simulink model "AsyncOnlinePlanning"  (R2025a)
settings: Solver=FixedStepAuto  StartTime=0.0  StopTime=inf  FixedStep=0.01  RelTol=1e-3  EnableMultiTasking=on
undefined symbols (not defined in the file): enable, finalPose, initialStateAndInput, originLLA, reset, samplingBoxCenterPose, samplingBoxDimension, sequentialPlanner, timestamp, verticesStaticObstacles
libraries: MPSV x4, simulink x2
settings Model: Creator=damerius  LastModifiedBy=damerius
settings SolverCC: ConcurrentTasks=on  AlgebraicLoopSolver=TrustRegion  PositivePriorityOrder=on
settings DataIOCC: SaveOutput=off  SignalLogging=off  DSMLogging=off  SaveTime=off  ReturnWorkspaceOutputs=off
settings OptimizationCC: DefaultParameterBehavior=Inlined  ReuseModelBlockBuffer=off  ZeroExternalMemoryAtStartup=off  ZeroInternalMemoryAtStartup=off  SimCompilerOptimization=on
settings DebuggingCC: UnconnectedInputMsg=warning  UnconnectedOutputMsg=warning  UnconnectedLineMsg=warning
settings HardwareCC: ProdBitPerLong=64.0  ProdHWDeviceType=Intel->x86-64 (Linux 64)
settings ModelReferenceCC: EnableRefExpFcnMdlSchedulingChecks=on
settings SFSimCC: SimParseCustomCode=off  SimGenImportedTypeDefs=on  SimTargetLang=C++  SimDLTargetLibrary=mkl-dnn
settings RTWCC: GenCodeOnly=on  PackageGeneratedCodeAndArtifacts=on  PackageName=PackNGo  RTWVerbose=off  BuildConfiguration=Faster Runs  TargetLang=C++  GPUComputeCapability=3.5  DLArmComputeVersion=19.05
settings CodeAppCC: ForceParamTrailComments=on  MaxIdLength=95.0  MATLABSourceComments=on  UseSimReservedNames=on
settings GRTTargetCC: TargetLangStandard=C++11 (ISO)  GenerateFullHeader=off  MatFileLogging=off  CodeInterfacePackaging=C++ class  SubcomponentCodeInterfacePackaging=C++ class

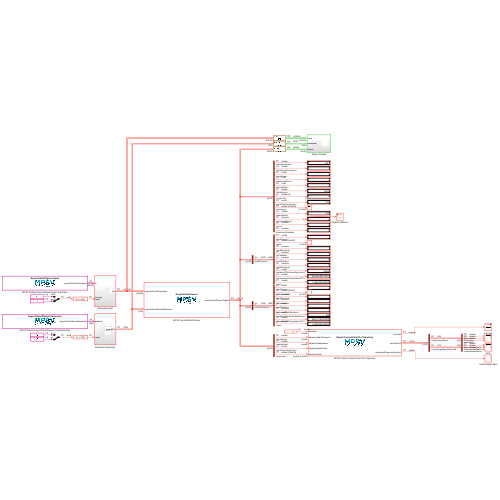
[thumbnail: Simulink's stored preview of the top-level diagram]
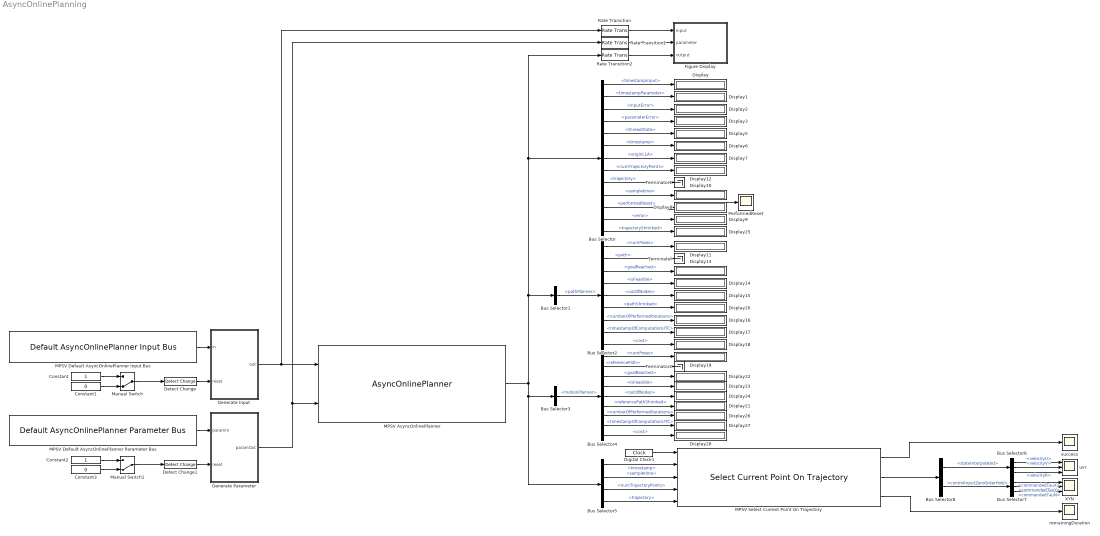
== system AsyncOnlinePlanning ==
  Bus Selector : BusSelector  OutputSignals=timestampInput,timestampParameter,inputError,parameterError,threadState,timestamp,originLLA,numTrajectoryPoints,trajectory,sampletime,performedReset,error,trajectoryShrinked
  Bus Selector1 : BusSelector  OutputSignals=pathPlanner
  Bus Selector2 : BusSelector  OutputSignals=numPoses,path,goalReached,isFeasible,outOfNodes,pathShrinked,numberOfPerformedIterations,timestampOfComputationUTC,cost
  Bus Selector3 : BusSelector  OutputSignals=motionPlanner
  Bus Selector4 : BusSelector  OutputSignals=numPoses,referencePath,goalReached,isFeasible,outOfNodes,referencePathShrinked,numberOfPerformedIterations,timestampOfComputationUTC,cost
  Bus Selector5 : BusSelector  OutputSignals=timestamp,sampletime,numTrajectoryPoints,trajectory
  Bus Selector6 : BusSelector  OutputSignals=velocityU,velocityV,velocityR
  Bus Selector7 : BusSelector  OutputSignals=commandedTauX,commandedTauY,commandedTauN
  Bus Selector8 : BusSelector  OutputSignals=stateInterpolated,controlInputZeroOrderHold
  Constant : Constant  OutDataTypeStr=uint8
  Constant1 : Constant  Value=0  OutDataTypeStr=uint8
  Constant2 : Constant  OutDataTypeStr=uint8
  Constant3 : Constant  Value=0  OutDataTypeStr=uint8
  Detect Change : simulink/Logic and Bit Operations/Detect Change  vinit=0  OutDataTypeStr=boolean
  Detect Change1 : simulink/Logic and Bit Operations/Detect Change  vinit=0  OutDataTypeStr=boolean
  Digital Clock1 : DigitalClock  SampleTime=0.01
  Display{,1..3,5..28} (28 alike) : Display
  Figure Display : Subsystem
  Generate Input : Subsystem
  Generate Parameter : Subsystem
  MPSV AsyncOnlinePlanner : MPSV/AsyncOnlinePlanner  pathMaxNumNodes=250  pathMaxNumSamples=1000000  motionMaxNumNodes=250  motionMaxNumSamples=1000000  threadPriority=20  cpuCoreIDs=[]  ompNumThreads=-1  ompDynamic=-1
      settings: SourceProductName=MPSV - Motion Planner for Surface Vehicles
  MPSV Default AsyncOnlinePlanner Input Bus : MPSV/Default AsyncOnlinePlanner Input Bus
      settings: SourceProductName=MPSV - Motion Planner for Surface Vehicles
  MPSV Default AsyncOnlinePlanner Parameter Bus : MPSV/Default AsyncOnlinePlanner Parameter Bus
      settings: SourceProductName=MPSV - Motion Planner for Surface Vehicles
  MPSV Select Current Point On Trajectory : MPSV/Select Current Point On Trajectory
      settings: SourceProductName=MPSV - Motion Planner for Surface Vehicles
  Manual Switch : ManualSwitch  CurrentSetting=0
  Manual Switch1 : ManualSwitch  CurrentSetting=0
  PerformedReset : Scope
      settings: ActiveDisplayYMinimum=-0.125  ActiveDisplayYMaximum=1.125
  Rate Transition : RateTransition  Deterministic=off  OutPortSampleTime=1
  Rate Transition1 : RateTransition  Deterministic=off  OutPortSampleTime=1
  Rate Transition2 : RateTransition  Deterministic=off  OutPortSampleTime=1
  Terminator : Terminator
  Terminator1 : Terminator
  Terminator2 : Terminator
  XYN : Scope  NumInputPorts=3
      settings: ActiveDisplayYMinimum=-501.70849  ActiveDisplayYMaximum=735.84406
  remainingDuration : Scope
      settings: ActiveDisplayYMinimum=-2.9925  ActiveDisplayYMaximum=26.9325
  success : Scope
      settings: ActiveDisplayYMinimum=-0.125  ActiveDisplayYMaximum=1.125
  uvr : Scope  NumInputPorts=3
      settings: ActiveDisplayYMinimum=-0.33623  ActiveDisplayYMaximum=0.74355  DataLoggingVariableName=ScopeData2
  wires:
  MPSV Default AsyncOnlinePlanner Parameter Bus/1 -> Generate Parameter/1(paramIn)
  MPSV Default AsyncOnlinePlanner Input Bus/1 -> Generate Input/1(in)
  MPSV AsyncOnlinePlanner/1 -> Bus Selector5/1, Bus Selector3/1, Rate Transition2/1, Bus Selector/1, Bus Selector1/1
  Bus Selector/1 -> Display/1  "<timestampInput>"
  Bus Selector/2 -> Display1/1  "<timestampParameter>"
  Bus Selector/6 -> Display6/1  "<timestamp>"
  Bus Selector/7 -> Display7/1  "<originLLA>"
  Bus Selector/5 -> Display5/1  "<threadState>"
  Bus Selector/12 -> Display9/1  "<error>"
  Bus Selector/11 -> PerformedReset/1, Display8/1  "<performedReset>"
  Generate Parameter/1(paramOut) -> Rate Transition1/1, MPSV AsyncOnlinePlanner/2
  Generate Input/1(out) -> Rate Transition/1, MPSV AsyncOnlinePlanner/1
  Bus Selector/10 -> Display10/1  "<sampletime>"
  Bus Selector1/1 -> Bus Selector2/1  "<pathPlanner>"
  Bus Selector2/1 -> Display11/1  "<numPoses>"
  Bus Selector2/3 -> Display13/1  "<goalReached>"
  Bus Selector2/4 -> Display14/1  "<isFeasible>"
  Bus Selector2/5 -> Display15/1  "<outOfNodes>"
  Bus Selector2/7 -> Display16/1  "<numberOfPerformedIterations>"
  Bus Selector2/8 -> Display17/1  "<timestampOfComputationUTC>"
  Bus Selector2/9 -> Display18/1  "<cost>"
  Bus Selector2/2 -> Terminator/1  "<path>"
  Bus Selector/8 -> Display12/1  "<numTrajectoryPoints>"
  Bus Selector/9 -> Terminator1/1  "<trajectory>"
  Bus Selector3/1 -> Bus Selector4/1  "<motionPlanner>"
  Bus Selector4/1 -> Display19/1  "<numPoses>"
  Bus Selector4/2 -> Terminator2/1  "<referencePath>"
  Bus Selector4/3 -> Display22/1  "<goalReached>"
  Bus Selector4/6 -> Display21/1  "<referencePathShrinked>"
  Bus Selector4/7 -> Display26/1  "<numberOfPerformedIterations>"
  Bus Selector4/5 -> Display24/1  "<outOfNodes>"
  Bus Selector4/4 -> Display23/1  "<isFeasible>"
  Bus Selector4/9 -> Display28/1  "<cost>"
  Bus Selector4/8 -> Display27/1  "<timestampOfComputationUTC>"
  Rate Transition/1 -> Figure Display/1(input)
  Rate Transition1/1 -> Figure Display/2(parameter)
  Rate Transition2/1 -> Figure Display/3(output)
  Digital Clock1/1 -> MPSV Select Current Point On Trajectory/1
  Bus Selector5/1 -> MPSV Select Current Point On Trajectory/2  "<timestamp>"
  Bus Selector5/2 -> MPSV Select Current Point On Trajectory/3  "<sampletime>"
  Bus Selector5/3 -> MPSV Select Current Point On Trajectory/4  "<numTrajectoryPoints>"
  Bus Selector5/4 -> MPSV Select Current Point On Trajectory/5  "<trajectory>"
  MPSV Select Current Point On Trajectory/1 -> success/1
  Bus Selector8/1 -> Bus Selector6/1  "<stateInterpolated>"
  Bus Selector8/2 -> Bus Selector7/1  "<controlInputZeroOrderHold>"
  Bus Selector6/1 -> uvr/1  "<velocityU>"
  Bus Selector6/2 -> uvr/2  "<velocityV>"
  Bus Selector6/3 -> uvr/3  "<velocityR>"
  Bus Selector7/1 -> XYN/1  "<commandedTauX>"
  Bus Selector7/2 -> XYN/2  "<commandedTauY>"
  Bus Selector7/3 -> XYN/3  "<commandedTauN>"
  Constant/1 -> Manual Switch/1
  Constant1/1 -> Manual Switch/2
  Manual Switch/1 -> Detect Change/1
  MPSV Select Current Point On Trajectory/2 -> Bus Selector8/1
  MPSV Select Current Point On Trajectory/3 -> remainingDuration/1
  Detect Change/1 -> Generate Input/2(reset)
  Manual Switch1/1 -> Detect Change1/1
  Constant3/1 -> Manual Switch1/2
  Constant2/1 -> Manual Switch1/1
  Detect Change1/1 -> Generate Parameter/2(reset)
  Bus Selector2/6 -> Display20/1  "<pathShrinked>"
  Bus Selector/13 -> Display25/1  "<trajectoryShrinked>"
  Bus Selector/3 -> Display2/1  "<inputError>"
  Bus Selector/4 -> Display3/1  "<parameterError>"

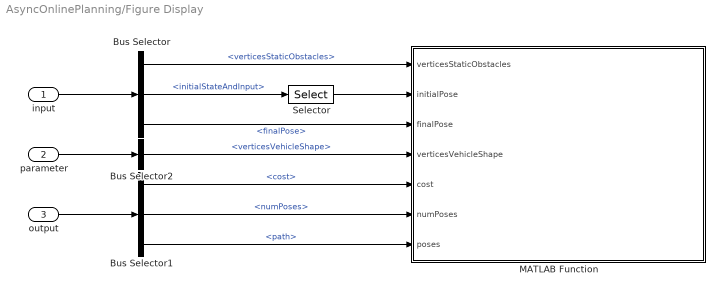
== system AsyncOnlinePlanning/Figure Display ==
  input : Inport
  parameter : Inport  Port=2
  output : Inport  Port=3
  Bus Selector : BusSelector  OutputSignals=verticesStaticObstacles,initialStateAndInput,finalPose
  Bus Selector1 : BusSelector  OutputSignals=pathPlanner.cost,pathPlanner.numPoses,pathPlanner.path
  Bus Selector2 : BusSelector  OutputSignals=sequentialPlanner.geometry.verticesVehicleShape
  MATLAB Function : MATLAB Function  TreatAsAtomicUnit=on
  Selector : Selector  InputPortWidth=12  IndexOptions=Index vector (dialog)  Indices=1:3  OutputSizes=1
  wires:
  Bus Selector2/1 -> MATLAB Function/4(verticesVehicleShape)  "<verticesVehicleShape>"
  Bus Selector1/3 -> MATLAB Function/7(poses)  "<path>"
  Bus Selector1/2 -> MATLAB Function/6(numPoses)  "<numPoses>"
  Bus Selector1/1 -> MATLAB Function/5(cost)  "<cost>"
  output/1 -> Bus Selector1/1
  Bus Selector/3 -> MATLAB Function/3(finalPose)  "<finalPose>"
  Bus Selector/2 -> Selector/1  "<initialStateAndInput>"
  Bus Selector/1 -> MATLAB Function/1(verticesStaticObstacles)  "<verticesStaticObstacles>"
  input/1 -> Bus Selector/1
  Selector/1 -> MATLAB Function/2(initialPose)
  parameter/1 -> Bus Selector2/1

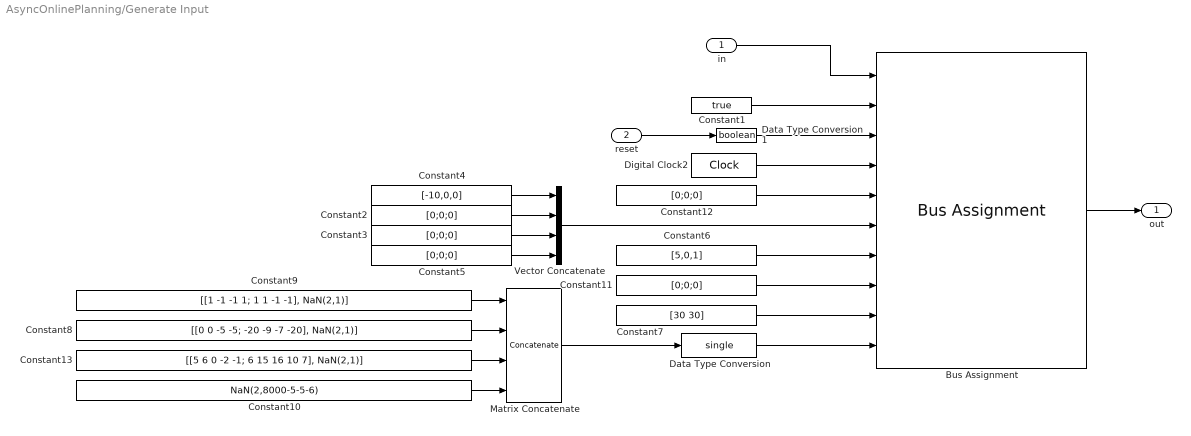
== system AsyncOnlinePlanning/Generate Input ==
  in : Inport
  reset : Inport  Port=2
  Bus Assignment : BusAssignment  AssignedSignals=enable,reset,timestamp,originLLA,initialStateAndInput,finalPose,samplingBoxCenterPose,samplingBoxDimension,verticesStaticObstacles
  Constant1 : Constant  Value=true  OutDataTypeStr=boolean
  Constant10 : Constant  Value=NaN(2,8000-5-5-6)
  Constant{2..3,5,11..12} (5 alike) : Constant  Value=[0;0;0]
  Constant13 : Constant  Value=[[5 6 0 -2 -1; 6 15 16 10 7], NaN(2,1)]
  Constant4 : Constant  Value=[-10,0,0]
  Constant6 : Constant  Value=[5,0,1]
  Constant7 : Constant  Value=[30 30]
  Constant8 : Constant  Value=[[0 0 -5 -5; -20 -9 -7 -20], NaN(2,1)]
  Constant9 : Constant  Value=[[1 -1 -1 1; 1 1 -1 -1], NaN(2,1)]
  Data Type Conversion : DataTypeConversion  OutDataTypeStr=single  SaturateOnIntegerOverflow=off  RndMeth=Floor
  Data Type Conversion1 : DataTypeConversion  OutDataTypeStr=boolean  SaturateOnIntegerOverflow=off  RndMeth=Floor
  Digital Clock2 : DigitalClock  SampleTime=0.01
  Matrix Concatenate : Concatenate  NumInputs=4  Mode=Multidimensional array  ConcatenateDimension=2
  Vector Concatenate : Concatenate  NumInputs=4
  out : Outport
  wires:
  in/1 -> Bus Assignment/1
  Bus Assignment/1 -> out/1
  reset/1 -> Data Type Conversion1/1
  Constant1/1 -> Bus Assignment/2
  Constant12/1 -> Bus Assignment/5
  Constant4/1 -> Vector Concatenate/1
  Constant2/1 -> Vector Concatenate/2
  Constant3/1 -> Vector Concatenate/3
  Constant5/1 -> Vector Concatenate/4
  Vector Concatenate/1 -> Bus Assignment/6
  Constant6/1 -> Bus Assignment/7
  Constant11/1 -> Bus Assignment/8
  Constant7/1 -> Bus Assignment/9
  Data Type Conversion1/1 -> Bus Assignment/3
  Digital Clock2/1 -> Bus Assignment/4
  Constant9/1 -> Matrix Concatenate/1
  Constant10/1 -> Matrix Concatenate/4
  Constant13/1 -> Matrix Concatenate/3
  Constant8/1 -> Matrix Concatenate/2
  Matrix Concatenate/1 -> Data Type Conversion/1
  Data Type Conversion/1 -> Bus Assignment/10

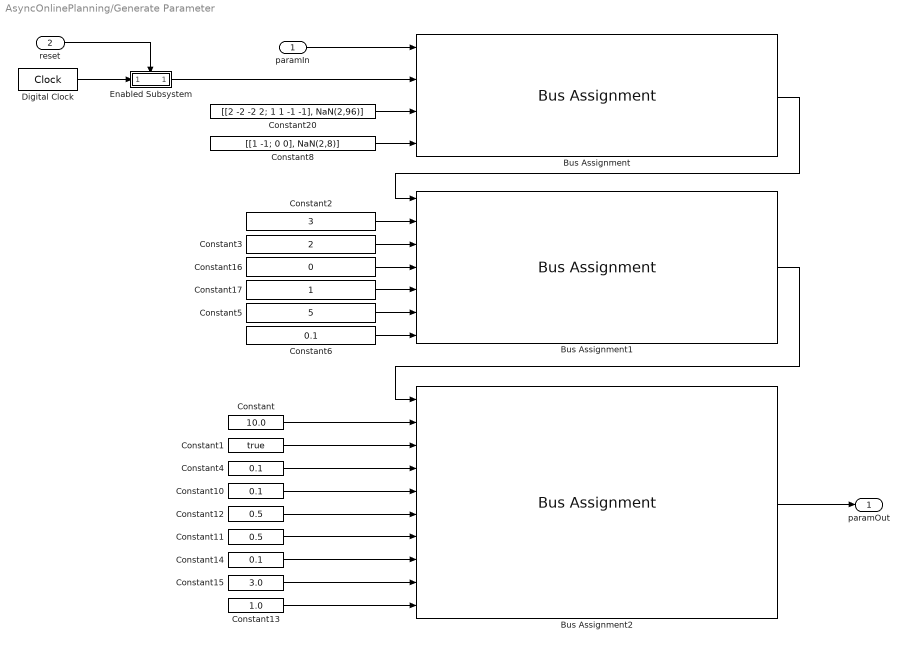
== system AsyncOnlinePlanning/Generate Parameter ==
  paramIn : Inport
  reset : Inport  Port=2
  Bus Assignment : BusAssignment  AssignedSignals=timestamp,sequentialPlanner.geometry.verticesVehicleShape,sequentialPlanner.geometry.skeletalPoints
  Bus Assignment1 : BusAssignment  AssignedSignals=sequentialPlanner.metric.weightPsi,sequentialPlanner.metric.weightSway,sequentialPlanner.metric.weightReverseScale,sequentialPlanner.metric.weightReverseDecay,sequentialPlanner.costMap.distanceScale,sequentialPlanner.costMap.distanceDecay
  Bus Assignment2 : BusAssignment  AssignedSignals=timeoutInput,onlinePlanner.predictInitialStateOnReset,onlinePlanner.maxComputationTimePathOnReset,onlinePlanner.maxComputationTimeMotionOnReset,onlinePlanner.maxComputationTimePath,onlinePlanner.maxComputationTimeMotion,onlinePlanner.additionalAheadPlanningTime,onlinePlanner.additionalTrajectoryDuration,onlinePlanner.timeKeepPastTrajectory
  Constant : Constant  Value=10.0  OutDataTypeStr=double
  Constant1 : Constant  Value=true  OutDataTypeStr=boolean
  Constant10 : Constant  Value=0.1  OutDataTypeStr=double
  Constant11 : Constant  Value=0.5  OutDataTypeStr=double
  Constant12 : Constant  Value=0.5  OutDataTypeStr=double
  Constant13 : Constant  Value=1.0  OutDataTypeStr=double
  Constant14 : Constant  Value=0.1  OutDataTypeStr=double
  Constant15 : Constant  Value=3.0  OutDataTypeStr=double
  Constant16 : Constant  Value=0
  Constant17 : Constant
  Constant2 : Constant  Value=3
  Constant20 : Constant  Value=[[2 -2 -2 2; 1 1 -1 -1], NaN(2,96)]  OutDataTypeStr=single
  Constant3 : Constant  Value=2
  Constant4 : Constant  Value=0.1  OutDataTypeStr=double
  Constant5 : Constant  Value=5
  Constant6 : Constant  Value=0.1
  Constant8 : Constant  Value=[[1 -1; 0 0], NaN(2,8)]  OutDataTypeStr=single
  Digital Clock : DigitalClock  SampleTime=0.01
  Enabled Subsystem : Subsystem  TreatAsAtomicUnit=on
  paramOut : Outport
  wires:
  paramIn/1 -> Bus Assignment/1
  Constant8/1 -> Bus Assignment/4
  Bus Assignment/1 -> Bus Assignment1/1
  Constant6/1 -> Bus Assignment1/7
  Constant5/1 -> Bus Assignment1/6
  Constant3/1 -> Bus Assignment1/3
  Constant2/1 -> Bus Assignment1/2
  Bus Assignment1/1 -> Bus Assignment2/1
  Bus Assignment2/1 -> paramOut/1
  Constant/1 -> Bus Assignment2/2
  Constant1/1 -> Bus Assignment2/3
  Constant4/1 -> Bus Assignment2/4
  Constant10/1 -> Bus Assignment2/5
  Constant11/1 -> Bus Assignment2/7
  Constant12/1 -> Bus Assignment2/6
  Constant13/1 -> Bus Assignment2/10
  Constant14/1 -> Bus Assignment2/8
  Constant15/1 -> Bus Assignment2/9
  Digital Clock/1 -> Enabled Subsystem/1(In1)
  Enabled Subsystem/1(time) -> Bus Assignment/2
  reset/1 -> Enabled Subsystem/Enable
  Constant16/1 -> Bus Assignment1/4
  Constant17/1 -> Bus Assignment1/5
  Constant20/1 -> Bus Assignment/3

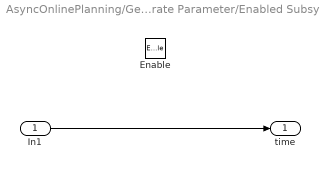
== system AsyncOnlinePlanning/Generate Parameter/Enabled Subsystem ==
  In1 : Inport
  Enable : EnablePort
  time : Outport
  wires:
  In1/1 -> time/1

== matlab function AsyncOnlinePlanning/Figure Display/MATLAB Function ==
  data: verticesStaticObstacles input; initialPose input; finalPose input; verticesVehicleShape input; cost input; numPoses input; poses input
function FigureDisplay(verticesStaticObstacles, initialPose, finalPose, verticesVehicleShape, cost, numPoses, poses)
    persistent f;
    if(isempty(f))
        f = figure(42);
    end

    clf;
    hold on;
    PlotPath(numPoses, poses, verticesVehicleShape, [0 0.3 0.5]);
    PlotVehicleShape(initialPose, verticesVehicleShape, [0.9 0 0]);
    PlotVehicleShape(finalPose, verticesVehicleShape, [0 0.7 0]);
    PlotObstacles(verticesStaticObstacles);
    view(90,-90);
    axis equal;
    box on;
    grid on;
    xlabel('x in m');
    ylabel('y in m');
    title(sprintf('cost: %f',cost));
    drawnow();
end

function PlotPath(numPoses, poses, verticesVehicleShape, color)
    x = poses(1,1:numPoses);
    y = poses(2,1:numPoses);
    plot(x,y,'LineWidth',2,'Color',color);
    for i = uint32(1):uint32(numPoses)
        PlotVehicleShape(poses(:,i), verticesVehicleShape, color);
    end
end

function PlotVehicleShape(pose, verticesVehicleShape, color)
    c = cos(pose(3));
    s = sin(pose(3));
    R = [c -s; s c];

    N = int32(size(verticesVehicleShape,2));
    i0 = int32(-1);

    for i = int32(1):N
        finiteVertex = isfinite(verticesVehicleShape(1,i)) && isfinite(verticesVehicleShape(2,i));
        if((i0 < 1) && finiteVertex)
            i0 = i;
        elseif((i0 > 0) && (~finiteVertex || (i == N)))
            i = i + int32((i == N) && finiteVertex);
            vertices = R * verticesVehicleShape(:,i0:(i-1)) + [pose(1); pose(2)];
            PlotPolygon(vertices, color);
            plot(pose(1),pose(2),'o','Color',color);
            i0 = int32(-1);
        end
    end
end

function PlotObstacles(verticesStaticObstacles)
    N = int32(size(verticesStaticObstacles,2));
    i0 = int32(-1);

    for i = int32(1):N
        finiteVertex = isfinite(verticesStaticObstacles(1,i)) && isfinite(verticesStaticObstacles(2,i));
        if((i0 < 1) && finiteVertex)
            i0 = i;
        elseif((i0 > 0) && (~finiteVertex || (i == N)))
            i = i + int32((i == N) && finiteVertex);
            PlotPolygon(verticesStaticObstacles(:,i0:(i-1)), [0,0,0]);
            i0 = int32(-1);
        end
    end
end

function PlotPolygon(vertices, color)
    x = [vertices(1,:) vertices(1,1)];
    y = [vertices(2,:) vertices(2,1)];
    plot(x,y,'LineWidth',1,'Color',color);
end
